simulink model "assignment5"  (R2021b)
settings: Solver=VariableStepAuto  StartTime=0.0  StopTime=10.0  RelTol=1e-3
settings Model: Creator=rcmas  LastModifiedBy=rcmas

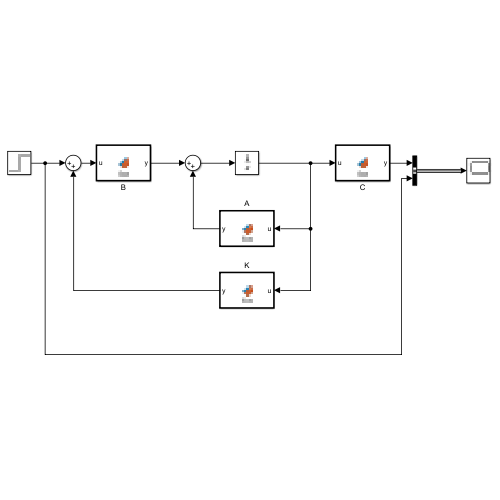
[thumbnail: Simulink's stored preview of the top-level diagram]
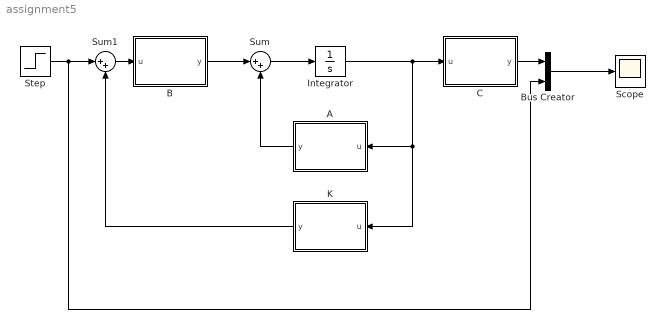
== system assignment5 ==
  A : MATLAB Function  TreatAsAtomicUnit=on
  B : MATLAB Function  TreatAsAtomicUnit=on
  Bus Creator : BusCreator  Inputs=2
  C : MATLAB Function  TreatAsAtomicUnit=on
  Integrator : Integrator  InitialCondition=[0;0]
  K : MATLAB Function  TreatAsAtomicUnit=on
  Scope : Scope
  Step : Step  Time=0  SampleTime=0
  Sum : Sum  Inputs=|++
  Sum1 : Sum  Inputs=|++
  wires:
  Integrator/1 -> K/1(u), A/1(u), C/1(u)
  Sum1/1 -> B/1(u)
  K/1(y) -> Sum1/2
  B/1(y) -> Sum/1
  A/1(y) -> Sum/2
  Sum/1 -> Integrator/1
  Step/1 -> Bus Creator/2, Sum1/1
  Bus Creator/1 -> Scope/1
  C/1(y) -> Bus Creator/1

== matlab function assignment5/C ==
  data: u input; y output
function y = fcn(u)
C=[ 1 0];
y = C*u;

== matlab function assignment5/A ==
  data: u input; y output
function y = fcn(u)
A=[0 1
    -3 -5];
y = A*u;

== matlab function assignment5/K ==
  data: u input; y output
function y = fcn(u)
K=-[180.1 11];
y = K*u;

== matlab function assignment5/B ==
  data: u input; y output
function y = fcn(u)
B=[0 ; 1];
y = B*u;
